simulink model "methode_asservissement"  (R2023b)
settings: Solver=VariableStepAuto  StartTime=0.0  StopTime=50  FixedStep=0.01  RelTol=1e-3
model workspace (MAT data in the model file):
  J = 1
undefined symbols (not defined in the file or in its folder): K
settings Model: Creator=alexi  LastModifiedBy=matth

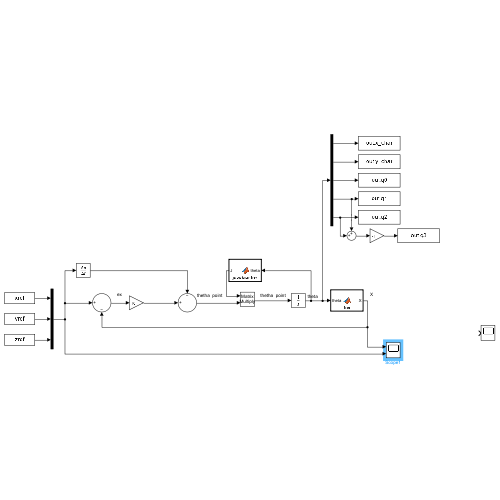
[thumbnail: Simulink's stored preview of the top-level diagram]
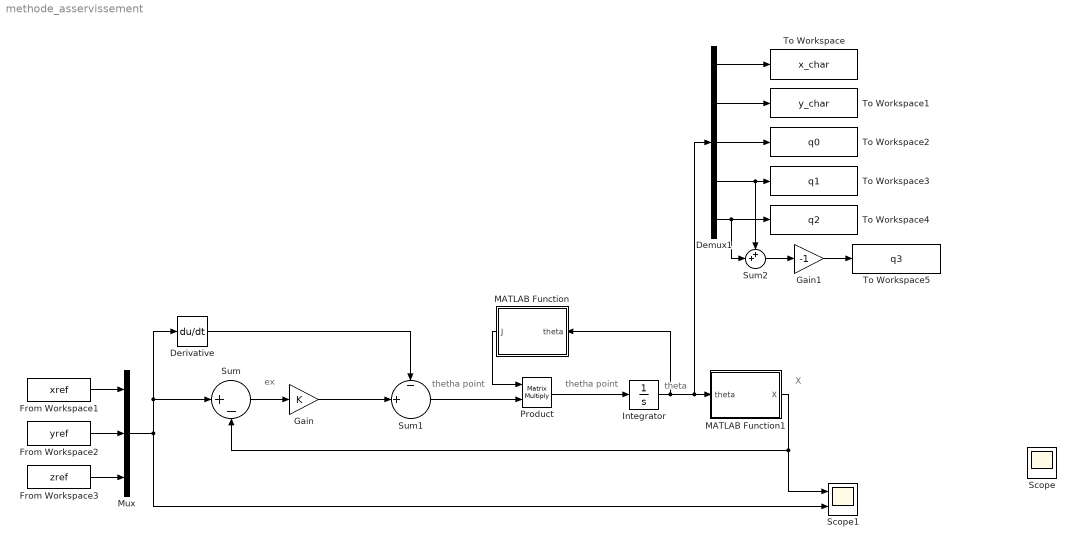
== system methode_asservissement ==
  note: ex
  note: X
  note: theta
  note: thetha point
  note: thetha point
  Demux1 : Demux  Outputs=5
  Derivative : Derivative
  From Workspace1 : FromWorkspace  VariableName=xref
  From Workspace2 : FromWorkspace  VariableName=yref
  From Workspace3 : FromWorkspace  VariableName=zref
  Gain : Gain  Gain=K
  Gain1 : Gain  Gain=-1
  Integrator : Integrator
  MATLAB Function : MATLAB Function  TreatAsAtomicUnit=on
  MATLAB Function1 : MATLAB Function  TreatAsAtomicUnit=on
  Mux : Mux  Inputs=3
  Product : Product  Multiplication=Matrix(*)
  Scope : Scope
  Scope1 : Scope  NumInputPorts=2
  Sum : Sum  Inputs=|+-
  Sum1 : Sum  Inputs=-|+||
  Sum2 : Sum  Inputs=++|
  To Workspace : ToWorkspace  VariableName=x_char  SaveFormat=Timeseries  SampleTime=-1
  To Workspace1 : ToWorkspace  VariableName=y_char  SaveFormat=Timeseries  SampleTime=-1
  To Workspace2 : ToWorkspace  VariableName=q0  SaveFormat=Timeseries  SampleTime=-1
  To Workspace3 : ToWorkspace  VariableName=q1  SaveFormat=Timeseries  SampleTime=-1
  To Workspace4 : ToWorkspace  VariableName=q2  SaveFormat=Timeseries  SampleTime=-1
  To Workspace5 : ToWorkspace  VariableName=q3  SaveFormat=Timeseries  SampleTime=-1
  wires:
  Sum/1 -> Gain/1
  Product/1 -> Integrator/1
  Gain/1 -> Sum1/2
  Derivative/1 -> Sum1/1
  Integrator/1 -> MATLAB Function/1(theta), Demux1/1, MATLAB Function1/1(theta)
  From Workspace3/1 -> Mux/3
  From Workspace1/1 -> Mux/1
  From Workspace2/1 -> Mux/2
  MATLAB Function/1(J) -> Product/1
  Sum1/1 -> Product/2
  Demux1/1 -> To Workspace/1
  Demux1/2 -> To Workspace1/1
  Demux1/3 -> To Workspace2/1
  Demux1/4 -> Sum2/1, To Workspace3/1
  Demux1/5 -> Sum2/2, To Workspace4/1
  Gain1/1 -> To Workspace5/1
  Sum2/1 -> Gain1/1
  MATLAB Function1/1(X) -> Sum/2, Scope1/1
  Mux/1 -> Derivative/1, Sum/1, Scope1/2

== matlab function methode_asservissement/MATLAB Function ==
  data: J output; theta input


function J = jacobianInv(theta)
    J = zeros(5, 3);
    theta0 = theta(3);
    theta1 = theta(4);
    theta2 = theta(5);
    D1 = 0.128;
    d1 = 0.024;
    D2 = 0.124;
    val1 = -D1*sin(theta1) + d1*cos(theta1) + D2*cos(theta1 + theta2);
    val2 = -D1*cos(theta1) - d1*sin(theta1) - D2*sin(theta1 + theta2);
    val3 = -D1*sin(theta1) + d1*cos(theta1) + D2*cos(theta1 + theta2);
    Jac = [1, 0, -sin(theta0)*val1, cos(theta0)*val2, -D2*sin(theta1 + theta2)*cos(theta0);
           0, 1, cos(theta0)*val1, sin(theta0)*val2, -D2*sin(theta1 + theta2)*sin(theta0) ;
           0, 0, 0, val3, D2*cos(theta1 + theta2)];
    J = pinv(Jac);
end

== matlab function methode_asservissement/MATLAB Function1 ==
  data: theta input; X output
function X = fcn(theta)
X = zeros(1, 3);

D0 = 0.077;
D1 = 0.128;
d1 = 0.024;
D2 = 0.124;
D3 = 0.126;

x = theta(1);
y = theta(2);
theta0 = theta(3);
theta1 = theta(4);
theta2 = theta(5);

X = [x + (-D1*sin(theta1) + d1*cos(theta1) + D2*cos(theta1 + theta2))*cos(theta0), y + (-D1*sin(theta1) + d1*cos(theta1) + D2*cos(theta1 + theta2))*sin(theta1), D0 + D1*cos(theta1) + d1*sin(theta1) + D2*sin(theta1 + theta2)];
end
